simulink model "Solve_Equation"  (R2022b)
settings: Solver=FixedStepAuto  StartTime=0.0  StopTime=10  RelTol=1e-3
settings Model: Creator=Dell  LastModifiedBy=Dell
settings OptimizationCC: DefaultParameterBehavior=Inlined  UseDivisionForNetSlopeComputation=on  GainParamInheritBuiltInType=on  UseFloatMulNetSlope=on  InlineInvariantSignals=on  PassReuseOutputArgsAs=Individual arguments  ZeroExternalMemoryAtStartup=off  ZeroInternalMemoryAtStartup=off  NoFixptDivByZeroProtection=on  EfficientFloat2IntCast=on  LifeSpan=1  OptimizeBlockOrder=speed  DifferentSizesBufferReuse=on  EfficientTunableParamExpr=on
settings DebuggingCC: ParameterTunabilityLossMsg=error
settings HardwareCC: ProdBitPerInt=16  ProdBitPerPointer=16  ProdBitPerSizeT=16  ProdBitPerPtrDiffT=16  ProdLargestAtomicFloat=None  ProdWordSize=8  ProdLongLongMode=on  ProdHWDeviceType=Atmel->AVR
settings SFSimCC: MATLABDynamicMemAlloc=off
settings RTWCC: Description=Embedded Coder  SystemTargetFile=ert.tlc  TemplateMakefile=ert_default_tmf
settings CodeAppCC: ForceParamTrailComments=on  IgnoreCustomStorageClasses=off  OperatorAnnotations=on  SimulinkDataObjDesc=on  SFDataObjDesc=on  CustomSymbolStrGlobalVar=rt$N$M  CustomSymbolStrType=$N$M  CustomSymbolStrFcn=$N$M$F  CustomSymbolStrMacro=$N$M  InsertBlockDesc=on
settings ERTTargetCC: TargetLangStandard=C99 (ISO)  GenerateSampleERTMain=on  IncludeMdlTerminateFcn=off  CombineSignalStateStructs=on  SupportAbsoluteTime=off  SupportComplex=off  SupportContinuousTime=on  InlinedParameterPlacement=NonHierarchical  ERTCustomFileTemplate=example_file_process.tlc  ERTFilePackagingFormat=CompactWithDataFile

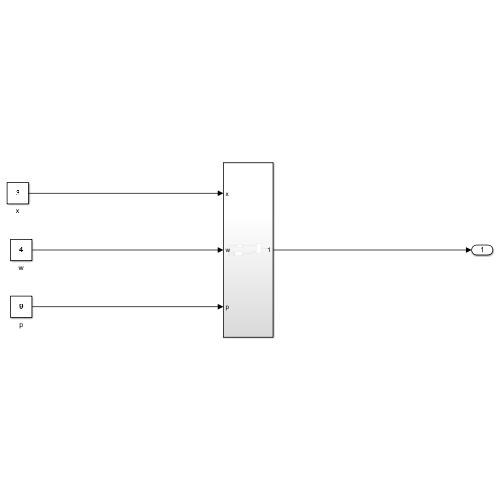
[thumbnail: Simulink's stored preview of the top-level diagram]
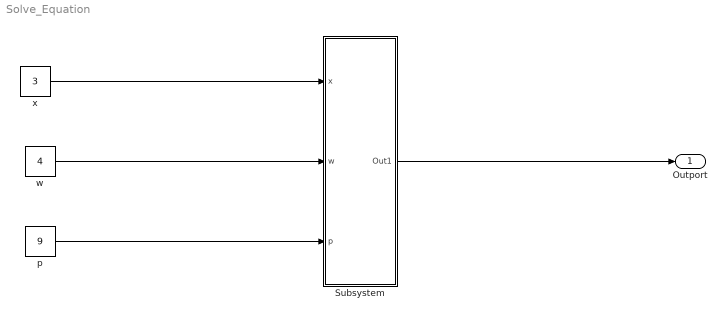
== system Solve_Equation ==
  Subsystem : Subsystem
  p : Constant  Value=9
  w : Constant  Value=4
  x : Constant  Value=3
  Outport : Outport
  wires:
  x/1 -> Subsystem/1(x)
  w/1 -> Subsystem/2(w)
  p/1 -> Subsystem/3(p)
  Subsystem/1(Out1) -> Outport/1

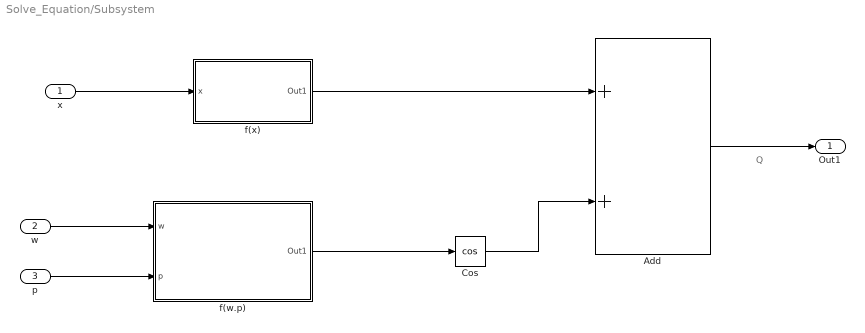
== system Solve_Equation/Subsystem ==
  note: Q
  x : Inport
  w : Inport  Port=2
  p : Inport  Port=3
  Add : Sum
  Cos : Trigonometry  Operator=cos
  f(w.p) : Subsystem
  f(x) : Subsystem
  Out1 : Outport
  wires:
  Cos/1 -> Add/2
  Add/1 -> Out1/1
  f(x)/1(Out1) -> Add/1
  f(w.p)/1(Out1) -> Cos/1
  w/1 -> f(w.p)/1(w)
  p/1 -> f(w.p)/2(p)
  x/1 -> f(x)/1(x)

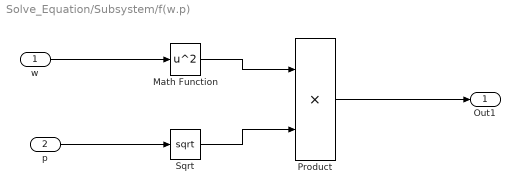
== system Solve_Equation/Subsystem/f(w.p) ==
  w : Inport
  p : Inport  Port=2
  Math Function : Math  Operator=square
  Product : Product
  Sqrt : Sqrt
  Out1 : Outport
  wires:
  Sqrt/1 -> Product/2
  Math Function/1 -> Product/1
  Product/1 -> Out1/1
  w/1 -> Math Function/1
  p/1 -> Sqrt/1

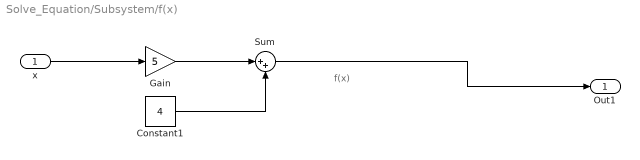
== system Solve_Equation/Subsystem/f(x) ==
  note: f(x)
  x : Inport
  Constant1 : Constant  Value=4
  Gain : Gain  Gain=5
  Sum : Sum  Inputs=|++
  Out1 : Outport
  wires:
  Constant1/1 -> Sum/2
  Sum/1 -> Out1/1
  x/1 -> Gain/1
  Gain/1 -> Sum/1
